simulink model "plotter_spring_damper"  (R2025a)
settings: Solver=VariableStepAuto  StartTime=0.0  StopTime=6  FixedStep=0.0001  MaxStep=1e-3  RelTol=1e-3
values from neighbouring files (symbols this model uses):
  alfa = cos(0.34906585)    [parameters.m]
  B_m = 0.000002    (= 2e-06)    [parameters.m]
  C = 3    [parameters.m]
  g = 9.8    [parameters.m]
  Gr = 1/30    (= 0.0333333333333)    [parameters.m]
  J_m = 0.000004    (= 4e-06)    [parameters.m]
  K = p_otimos(1)    [aproxima_segunda_ordem.m]    (also in motor_param.m = 23.26; parameters.m = 2040; valores_bruno.m = 23.26)
  K_t = 0.009    [parameters.m]
  L = 0.3    [cinematic_sim.m]    (also in parameters.m)
  L_a = 0.0023    [parameters.m]
  m = 0.1    [parameters.m]
  R = 0.017    [parameters.m]
  R_a = 2.182    [parameters.m]
libraries: slpidlib x2
settings Model: SimulationMode=accelerator  Creator=bruno  LastModifiedBy=bruno

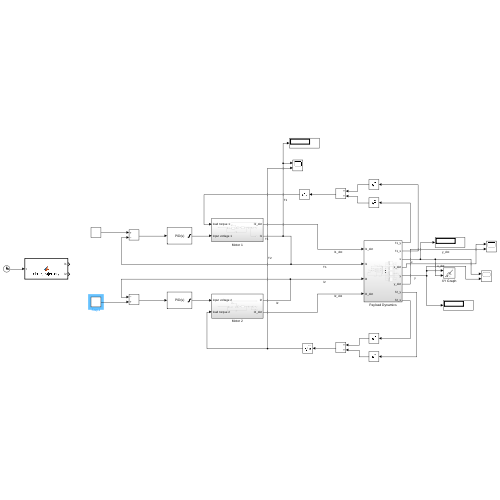
[thumbnail: Simulink's stored preview of the top-level diagram]
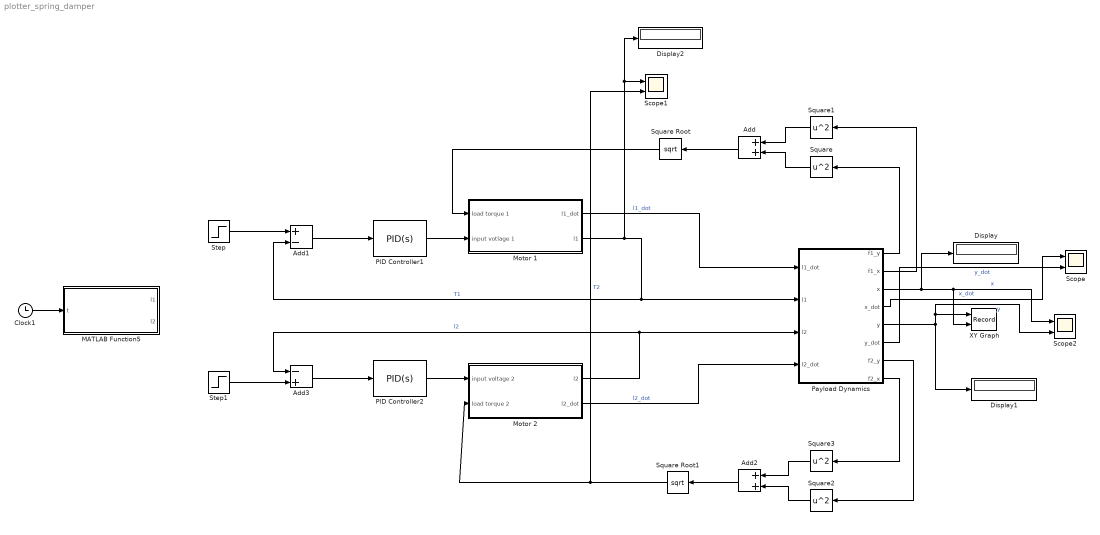
== system plotter_spring_damper ==
  Add : Sum
  Add1 : Sum  Inputs=+-
  Add2 : Sum
  Add3 : Sum  Inputs=-+
  Clock1 : Clock
      settings: Decimation=1000
  Display : Display
  Display1 : Display
  Display2 : Display
  MATLAB Function5 : MATLAB Function  TreatAsAtomicUnit=on
  Motor 1 : Subsystem
  Motor 2 : Subsystem
  PID Controller1 : slpidlib/PID Controller  Controller=PID  Form=Parallel  TimeDomain=Continuous-time  UseExternalTs=off  SampleTime=-1  IntegratorMethod=Forward Euler  FilterMethod=Forward Euler  ControllerParametersSource=internal  P=5109.01806071816  I=6474.67483762337  UseKiTs=off  D=175.0621895201  UseExternalDerivativeSource=off  N=17340.6505292231  UseFilter=on  TunerSelectOption=Transfer Function Based (PID Tuner App)  InitialConditionSource=internal  InitialConditionForIntegrator=0  InitialConditionForFilter=0  DifferentiatorICPrevScaledInput=0  ExternalReset=none  TrackingMode=off  Kt=1  LimitOutput=on  SatLimitsSource=internal  UpperSaturationLimit=12  LowerSaturationLimit=-12  LinearizeAsGain=on  AntiWindupMode=none  Kb=1  LimitIntegrator=off  UpperIntegratorSaturationLimit=inf  LowerIntegratorSaturationLimit=-inf  POutMin=[]  POutMax=[]  IOutMin=[]  IOutMax=[]  DOutMin=[]  DOutMax=[]  NOutMin=[]  NOutMax=[]  SumOutMin=[]  SumOutMax=[]  SaturationOutMin=[]  SaturationOutMax=[]  PParamMin=[]  PParamMax=[]  IParamMin=[]  IParamMax=[]  DParamMin=[]  DParamMax=[]  NParamMin=[]  NParamMax=[]  KbParamMin=[]  KbParamMax=[]  KtParamMin=[]  KtParamMax=[]  KbOutMin=[]  KbOutMax=[]  KtOutMin=[]  KtOutMax=[]  IntegratorOutMin=[]  IntegratorOutMax=[]  FilterOutMin=[]  FilterOutMax=[]  SumI1OutMin=[]  SumI1OutMax=[]  SumI2OutMin=[]  SumI2OutMax=[]  SumI3OutMin=[]  SumI3OutMax=[]  SumI4OutMin=[]  SumI4OutMax=[]  SumDOutMin=[]  SumDOutMax=[]  DifferentiatorOutMin=[]  DifferentiatorOutMax=[]  FilterDiffOutCoefMin=[]  FilterDiffOutCoefMax=[]  ReciprocalOutMin=[]  ReciprocalOutMax=[]  SumDenOutMin=[]  SumDenOutMax=[]  SumNumOutMin=[]  SumNumOutMax=[]  DivideOutMin=[]  DivideOutMax=[]  UdiffTsProdOutMin=[]  UdiffTsProdOutMax=[]  NTsProdOutMin=[]  NTsProdOutMax=[]  UintegralTsProdOutMin=[]  UintegralTsProdOutMax=[]  UngainTsProdOutMin=[]  UngainTsProdOutMax=[]  ClampingZeroOutDataTypeStr=Inherit: Inherit via back propagation  ClampingZeroOutMin=[]  ClampingZeroOutMax=[]  FilterDenConstantOutDataTypeStr=Inherit: Inherit via back propagation  FilterDenConstantOutMin=[]  FilterDenConstantOutMax=[]  PCopyOutDataTypeStr=Inherit: Inherit via back propagation  PCopyOutMin=[]  PCopyOutMax=[]  NCopyOutDataTypeStr=Inherit: Inherit via back propagation  NCopyOutMin=[]  NCopyOutMax=[]  IntegratorContinuousStateAttributes=''  IntegratorStateMustResolveToSignalObject=off  IntegratorRTWStateStorageClass=Auto  FilterContinuousStateAttributes=''  FilterStateMustResolveToSignalObject=off  FilterRTWStateStorageClass=Auto  ParallelPVariant=InternalParameters  IdealPVariant=Disabled  IVariant=InternalParameters  DVariant=InternalParameters  IntegratorVariant=Continuous  SatVariant=Enabled  AWVariant=Passthrough  PCopyVariant=Disabled  TRVariant=Disabled  FdbkBlocksVariant=Forward  IdealPFdbkVariant=Disabled  SatFdbkVariant=Disabled  DerivativeFilterVariant=ContFilter  NVariant=InternalParameters  NCopyVariant=Disabled  FilterICVariant=InternalICsFilter  IntegratorICVariant=InternalICs  ExternalResetVariant=Disabled  TRSumVariant=Passthrough  SumFdbkVariant=Disabled  SumVariant=Sum_PID  TsampFilterVariant=InternalTs  TsampNgainVariant=Passthrough  TsampIntegralVariant=Disabled_SignalSpec  ExternalSaturationOutDataTypeStr=Inherit: Same as second input  DerivativeSourceVariant=ErrorSignal  PreIntVariant=InternalPreInt
  PID Controller2 : slpidlib/PID Controller  Controller=PID  Form=Parallel  TimeDomain=Continuous-time  UseExternalTs=off  SampleTime=-1  IntegratorMethod=Forward Euler  FilterMethod=Forward Euler  ControllerParametersSource=internal  P=5109.01806071816  I=6474.67483762337  UseKiTs=off  D=175.0621895201  UseExternalDerivativeSource=off  N=17340.6505292231  UseFilter=on  TunerSelectOption=Transfer Function Based (PID Tuner App)  InitialConditionSource=internal  InitialConditionForIntegrator=0  InitialConditionForFilter=0  DifferentiatorICPrevScaledInput=0  ExternalReset=none  TrackingMode=off  Kt=1  LimitOutput=on  SatLimitsSource=internal  UpperSaturationLimit=12  LowerSaturationLimit=-12  LinearizeAsGain=on  AntiWindupMode=none  Kb=1  LimitIntegrator=off  UpperIntegratorSaturationLimit=inf  LowerIntegratorSaturationLimit=-inf  POutMin=[]  POutMax=[]  IOutMin=[]  IOutMax=[]  DOutMin=[]  DOutMax=[]  NOutMin=[]  NOutMax=[]  SumOutMin=[]  SumOutMax=[]  SaturationOutMin=[]  SaturationOutMax=[]  PParamMin=[]  PParamMax=[]  IParamMin=[]  IParamMax=[]  DParamMin=[]  DParamMax=[]  NParamMin=[]  NParamMax=[]  KbParamMin=[]  KbParamMax=[]  KtParamMin=[]  KtParamMax=[]  KbOutMin=[]  KbOutMax=[]  KtOutMin=[]  KtOutMax=[]  IntegratorOutMin=[]  IntegratorOutMax=[]  FilterOutMin=[]  FilterOutMax=[]  SumI1OutMin=[]  SumI1OutMax=[]  SumI2OutMin=[]  SumI2OutMax=[]  SumI3OutMin=[]  SumI3OutMax=[]  SumI4OutMin=[]  SumI4OutMax=[]  SumDOutMin=[]  SumDOutMax=[]  DifferentiatorOutMin=[]  DifferentiatorOutMax=[]  FilterDiffOutCoefMin=[]  FilterDiffOutCoefMax=[]  ReciprocalOutMin=[]  ReciprocalOutMax=[]  SumDenOutMin=[]  SumDenOutMax=[]  SumNumOutMin=[]  SumNumOutMax=[]  DivideOutMin=[]  DivideOutMax=[]  UdiffTsProdOutMin=[]  UdiffTsProdOutMax=[]  NTsProdOutMin=[]  NTsProdOutMax=[]  UintegralTsProdOutMin=[]  UintegralTsProdOutMax=[]  UngainTsProdOutMin=[]  UngainTsProdOutMax=[]  ClampingZeroOutDataTypeStr=Inherit: Inherit via back propagation  ClampingZeroOutMin=[]  ClampingZeroOutMax=[]  FilterDenConstantOutDataTypeStr=Inherit: Inherit via back propagation  FilterDenConstantOutMin=[]  FilterDenConstantOutMax=[]  PCopyOutDataTypeStr=Inherit: Inherit via back propagation  PCopyOutMin=[]  PCopyOutMax=[]  NCopyOutDataTypeStr=Inherit: Inherit via back propagation  NCopyOutMin=[]  NCopyOutMax=[]  IntegratorContinuousStateAttributes=''  IntegratorStateMustResolveToSignalObject=off  IntegratorRTWStateStorageClass=Auto  FilterContinuousStateAttributes=''  FilterStateMustResolveToSignalObject=off  FilterRTWStateStorageClass=Auto  ParallelPVariant=InternalParameters  IdealPVariant=Disabled  IVariant=InternalParameters  DVariant=InternalParameters  IntegratorVariant=Continuous  SatVariant=Enabled  AWVariant=Passthrough  PCopyVariant=Disabled  TRVariant=Disabled  FdbkBlocksVariant=Forward  IdealPFdbkVariant=Disabled  SatFdbkVariant=Disabled  DerivativeFilterVariant=ContFilter  NVariant=InternalParameters  NCopyVariant=Disabled  FilterICVariant=InternalICsFilter  IntegratorICVariant=InternalICs  ExternalResetVariant=Disabled  TRSumVariant=Passthrough  SumFdbkVariant=Disabled  SumVariant=Sum_PID  TsampFilterVariant=InternalTs  TsampNgainVariant=Passthrough  TsampIntegralVariant=Disabled_SignalSpec  ExternalSaturationOutDataTypeStr=Inherit: Same as second input  DerivativeSourceVariant=ErrorSignal  PreIntVariant=InternalPreInt
  Payload Dynamics : Subsystem
  Scope : Scope  NumInputPorts=2
      settings: ActiveDisplayYMinimum=-0.62327143885854985  ActiveDisplayYMaximum=0.35966972632216176
  Scope1 : Scope  NumInputPorts=2
      settings: ActiveDisplayYMinimum=-0.38341696076365567  ActiveDisplayYMaximum=3.450752646872902  DataLoggingVariableName=ScopeData2
  Scope2 : Scope  NumInputPorts=2
      settings: ActiveDisplayYMinimum=0.20131924623409117  ActiveDisplayYMaximum=0.42229314319938704  DataLoggingVariableName=ScopeData3
  Square{,1..3} (4 alike) : Math  Operator=square
  Square Root : Sqrt
  Square Root1 : Sqrt
  Step : Step  Time=0  After=0.43  SampleTime=0
  Step1 : Step  Time=0  After=0.36  SampleTime=0
  XY Graph : Record  NumPorts=2.0  FileSettingsInternal="{\"entries\":[{\"content\":{\"excelSettings\":{\"content\":{},\"type\":\"Streamout.ExcelSettings\"},\"parquetSettings\":{\"content\":{},\"type\":\"Streamout.ParquetSettings\"}},\"type\":\"Streamout.FileSettingStorage\",\"uuid\":\"\"}],\"packageUris\":[\"http:\\/\\/schema.mathworks.com\\/mf0\\/streamout_blocks\\/R2020a\"],\"version\":\"1.0\"}"  FrameSettings=[0, 0]  Layout=[1 1]  SignalsInternal="{\"entries\":[{\"content\":{\"signals\":[{\"content\":{\"blockPath\":[],\"dimensions\":[1],\"domain\":\"\",\"lineColor\":\"#a2142f\",\"plots\":[ 1 ],\"port\":1,\"signalID\":1,\"signalName\":\"y\"},\"type\":\"RecordBlkView.Signal\",\"uuid\":\"\"},{\"content\":{\"blockPath\":[],\"dimensions\":[1],\"domain\":\"\",\"lineColor\":\"#139fff\",\"plots\":[ 1 ],\"port\":2,\"signalID\":2,\"signalName\":\"x\"},\"type\":\"RecordBlkView.Signal\",\"uuid\":\"\"}]},\"type\":\"RecordBlkView.InputSignals\",\"uuid\":\"\"}],\"packageUris\":[\"http:\\/\\/schema.mathworks.com\\/mf0\\/streamout_blocks\\/R2020a\"],\"version\":\"1.0\"}"  VisualizationBindings="{\"xyplotplugin\":{\"info\":[{\"series\":[{\"bindingParametersList\":[{\"parameter\":\"X-Axis\",\"signalID\":1,\"signalName\":\"y\"},{\"parameter\":\"Y-Axis\",\"signalID\":2,\"signalName\":\"x\"}],\"seriesID\":0}],\"subplotID\":1}]}}"  CompatibilityTag=XY
  wires:
  Square1/1 -> Add/1
  Square/1 -> Add/2
  Add/1 -> Square Root/1
  Square2/1 -> Add2/2
  Add2/1 -> Square Root1/1
  Square3/1 -> Add2/1
  PID Controller2/1 -> Motor 2/1(input voltage 2)
  PID Controller1/1 -> Motor 1/2(input votlage 1)
  Payload Dynamics/8(f2_x) -> Square3/1
  Payload Dynamics/7(f2_y) -> Square2/1
  Add1/1 -> PID Controller1/1
  Add3/1 -> PID Controller2/1
  Payload Dynamics/2(f1_x) -> Square1/1
  Payload Dynamics/3(x) -> XY Graph/2, Scope2/1, Display/1  "x"
  Payload Dynamics/5(y) -> XY Graph/1, Scope2/2, Display1/1  "y"
  Payload Dynamics/1(f1_y) -> Square/1
  Motor 1/1(l1_dot) -> Payload Dynamics/1(l1_dot)  "l1_dot"
  Motor 1/2(l1) -> Display2/1, Scope1/1, Add1/2, Payload Dynamics/2(l1)  "T1"
  Motor 2/2(l2_dot) -> Payload Dynamics/4(l2_dot)  "l2_dot"
  Square Root/1 -> Motor 1/1(load torque 1)
  Square Root1/1 -> Scope1/2, Motor 2/2(load torque 2)  "T2"
  Motor 2/1(l2) -> Add3/1, Payload Dynamics/3(l2)  "l2"
  Clock1/1 -> MATLAB Function5/1(t)
  Payload Dynamics/4(x_dot) -> Scope/1  "x_dot"
  Payload Dynamics/6(y_dot) -> Scope/2  "y_dot"
  Step/1 -> Add1/1
  Step1/1 -> Add3/2

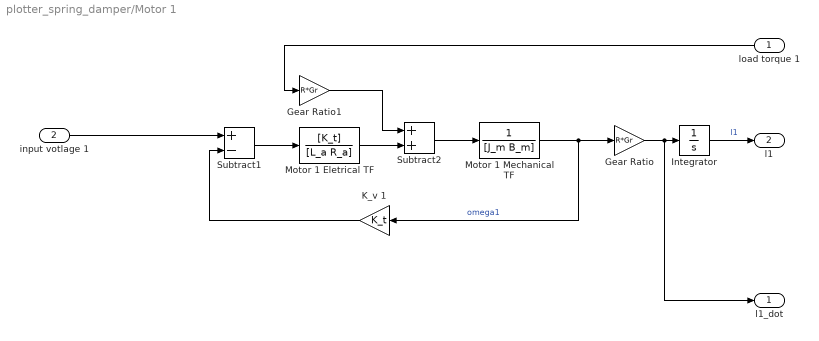
== system plotter_spring_damper/Motor 1 ==
  load torque 1 : Inport
  input votlage 1 : Inport  Port=2
  Gear Ratio : Gain  Gain=R*Gr
  Gear Ratio1 : Gain  Gain=R*Gr
  Integrator : Integrator  InitialCondition=0.461411
  K_v 1 : Gain  Gain=K_t
  Motor 1 Eletrical TF : TransferFcn  Numerator=[K_t]  Denominator=[L_a R_a]
  Motor 1 Mechanical TF : TransferFcn  Denominator=[J_m B_m]
  Subtract1 : Sum  Inputs=+-
  Subtract2 : Sum
  l1_dot : Outport
  l1 : Outport  Port=2
  wires:
  Motor 1 Eletrical TF/1 -> Subtract2/2
  load torque 1/1 -> Gear Ratio1/1
  K_v 1/1 -> Subtract1/2
  Gear Ratio1/1 -> Subtract2/1
  Subtract1/1 -> Motor 1 Eletrical TF/1
  Subtract2/1 -> Motor 1 Mechanical TF/1
  input votlage 1/1 -> Subtract1/1
  Motor 1 Mechanical TF/1 -> K_v 1/1, Gear Ratio/1  "omega1"
  Gear Ratio/1 -> l1_dot/1, Integrator/1
  Integrator/1 -> l1/1  "l1"

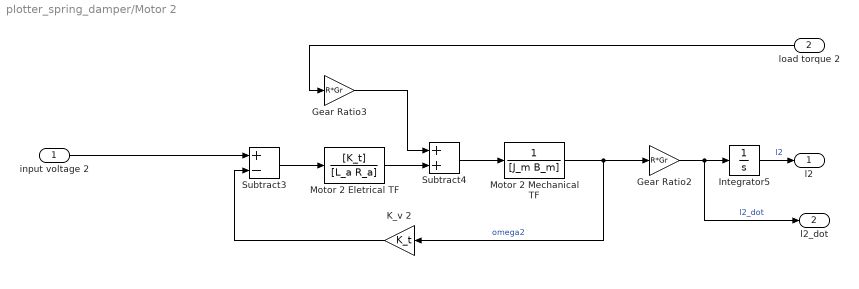
== system plotter_spring_damper/Motor 2 ==
  input voltage 2 : Inport
  load torque 2 : Inport  Port=2
  Gear Ratio2 : Gain  Gain=R*Gr
  Gear Ratio3 : Gain  Gain=R*Gr
  Integrator5 : Integrator  InitialCondition=0.406079
  K_v 2 : Gain  Gain=K_t
  Motor 2 Eletrical TF : TransferFcn  Numerator=[K_t]  Denominator=[L_a R_a]
  Motor 2 Mechanical TF : TransferFcn  Denominator=[J_m B_m]
  Subtract3 : Sum  Inputs=+-
  Subtract4 : Sum
  l2 : Outport
  l2_dot : Outport  Port=2
  wires:
  input voltage 2/1 -> Subtract3/1
  Motor 2 Eletrical TF/1 -> Subtract4/2
  Integrator5/1 -> l2/1  "l2"
  Subtract3/1 -> Motor 2 Eletrical TF/1
  Gear Ratio3/1 -> Subtract4/1
  Subtract4/1 -> Motor 2 Mechanical TF/1
  load torque 2/1 -> Gear Ratio3/1
  K_v 2/1 -> Subtract3/2
  Gear Ratio2/1 -> l2_dot/1, Integrator5/1  "l2_dot"
  Motor 2 Mechanical TF/1 -> Gear Ratio2/1, K_v 2/1  "omega2"

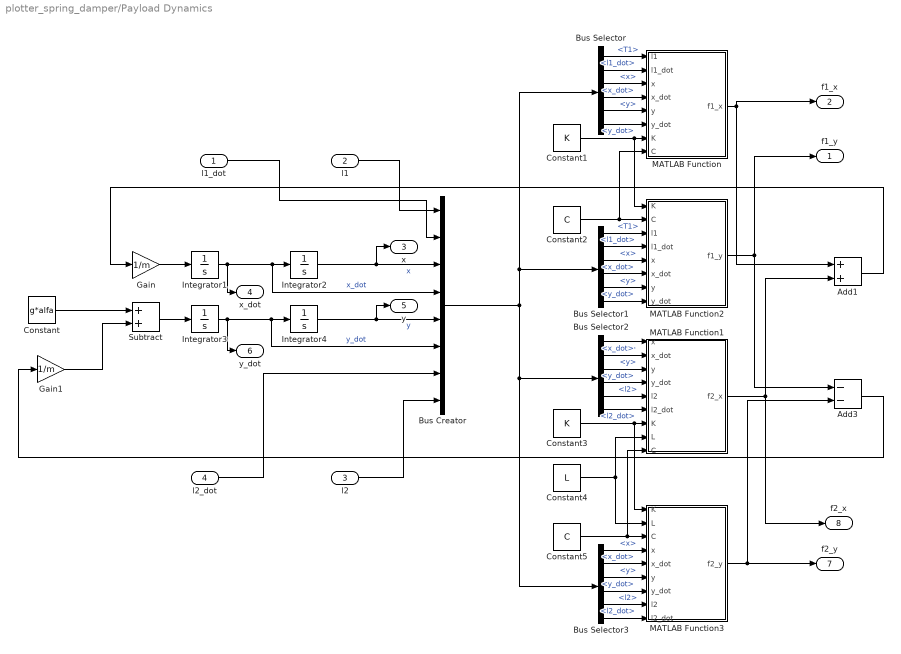
== system plotter_spring_damper/Payload Dynamics ==
  l1_dot : Inport
  l1 : Inport  Port=2
  l2 : Inport  Port=3
  l2_dot : Inport  Port=4
  Add1 : Sum
  Add3 : Sum  Inputs=--
  Bus Creator : BusCreator  Inputs=8
  Bus Selector : BusSelector  OutputSignals=T1,l1_dot,x,x_dot,y,y_dot
  Bus Selector1 : BusSelector  OutputSignals=T1,l1_dot,x,x_dot,y,y_dot
  Bus Selector2 : BusSelector  OutputSignals=x,x_dot,y,y_dot,l2,l2_dot
  Bus Selector3 : BusSelector  OutputSignals=x,x_dot,y,y_dot,l2,l2_dot
  Constant : Constant  Value=g*alfa
  Constant1 : Constant  Value=K
  Constant2 : Constant  Value=C
  Constant3 : Constant  Value=K
  Constant4 : Constant  Value=L
  Constant5 : Constant  Value=C
  Gain : Gain  Gain=1/m
  Gain1 : Gain  Gain=1/m
  Integrator1 : Integrator
  Integrator2 : Integrator  InitialCondition=0.23
  Integrator3 : Integrator
  Integrator4 : Integrator  InitialCondition=0.4
  MATLAB Function : MATLAB Function  TreatAsAtomicUnit=on
  MATLAB Function1 : MATLAB Function  TreatAsAtomicUnit=on
  MATLAB Function2 : MATLAB Function  TreatAsAtomicUnit=on
  MATLAB Function3 : MATLAB Function  TreatAsAtomicUnit=on
  Subtract : Sum
  f1_y : Outport
  f1_x : Outport  Port=2
  x : Outport  Port=3
  x_dot : Outport  Port=4
  y : Outport  Port=5
  y_dot : Outport  Port=6
  f2_y : Outport  Port=7
  f2_x : Outport  Port=8
  wires:
  Bus Selector1/2 -> MATLAB Function2/4(l1_dot)  "<l1_dot>"
  Bus Selector1/1 -> MATLAB Function2/3(l1)  "<T1>"
  Add3/1 -> Gain1/1
  Bus Selector1/6 -> MATLAB Function2/8(y_dot)  "<y_dot>"
  Constant3/1 -> MATLAB Function3/1(K), MATLAB Function1/7(K)
  Bus Selector1/4 -> MATLAB Function2/6(x_dot)  "<x_dot>"
  Bus Selector/4 -> MATLAB Function/4(x_dot)  "<x_dot>"
  Bus Selector/2 -> MATLAB Function/2(l1_dot)  "<l1_dot>"
  Bus Selector/1 -> MATLAB Function/1(l1)  "<T1>"
  Bus Selector/6 -> MATLAB Function/6(y_dot)  "<y_dot>"
  Bus Selector/3 -> MATLAB Function/3(x)  "<x>"
  Bus Selector/5 -> MATLAB Function/5(y)  "<y>"
  Integrator1/1 -> Bus Creator/4, Integrator2/1, x_dot/1  "x_dot"
  Constant/1 -> Subtract/1
  Bus Selector2/5 -> MATLAB Function1/5(l2)  "<l2>"
  Constant5/1 -> MATLAB Function3/3(C), MATLAB Function1/9(C)
  Integrator3/1 -> y_dot/1, Bus Creator/6, Integrator4/1  "y_dot"
  Bus Selector3/1 -> MATLAB Function3/4(x)  "<x>"
  Bus Selector3/3 -> MATLAB Function3/6(y)  "<y>"
  Constant4/1 -> MATLAB Function1/8(L), MATLAB Function3/2(L)
  Add1/1 -> Gain/1
  l1_dot/1 -> Bus Creator/2
  MATLAB Function/1(f1_x) -> Add1/1, f1_x/1
  l2_dot/1 -> Bus Creator/7
  l2/1 -> Bus Creator/8
  Bus Selector2/3 -> MATLAB Function1/3(y)  "<y>"
  Constant1/1 -> MATLAB Function2/1(K), MATLAB Function/7(K)
  l1/1 -> Bus Creator/1
  MATLAB Function3/1(f2_y) -> Add3/2, f2_y/1
  Gain/1 -> Integrator1/1
  Bus Selector2/1 -> MATLAB Function1/1(x)  "<x>"
  MATLAB Function1/1(f2_x) -> f2_x/1, Add1/2
  Bus Selector2/2 -> MATLAB Function1/2(x_dot)  "<x_dot>"
  Bus Selector3/6 -> MATLAB Function3/9(l2_dot)  "<l2_dot>"
  Integrator4/1 -> y/1, Bus Creator/5  "y"
  Bus Selector2/4 -> MATLAB Function1/4(y_dot)  "<y_dot>"
  Integrator2/1 -> x/1, Bus Creator/3  "x"
  Bus Creator/1 -> Bus Selector3/1, Bus Selector2/1, Bus Selector1/1, Bus Selector/1
  Bus Selector3/5 -> MATLAB Function3/8(l2)  "<l2>"
  MATLAB Function2/1(f1_y) -> f1_y/1, Add3/1
  Bus Selector3/4 -> MATLAB Function3/7(y_dot)  "<y_dot>"
  Bus Selector3/2 -> MATLAB Function3/5(x_dot)  "<x_dot>"
  Constant2/1 -> MATLAB Function2/2(C), MATLAB Function/8(C)
  Subtract/1 -> Integrator3/1
  Bus Selector1/3 -> MATLAB Function2/5(x)  "<x>"
  Bus Selector1/5 -> MATLAB Function2/7(y)  "<y>"
  Gain1/1 -> Subtract/2
  Bus Selector2/6 -> MATLAB Function1/6(l2_dot)  "<l2_dot>"

== matlab function plotter_spring_damper/Payload Dynamics/MATLAB Function1 ==
  data: x input; x_dot input; f2_x output; y input; y_dot input; l2 input; l2_dot input; K input; L input; C input
function f2_x = F2_x(x,x_dot,y,y_dot,l2,l2_dot,K,L,C)
    distance2 = sqrt((L-x)^2 + y^2);
    if distance2 > l2 
        f2_x = (K*(distance2 -l2) + C*((x*x_dot -L*x_dot + y*y_dot)/distance2 - l2_dot))*(L-x)/distance2;
    else
        f2_x = 0;
    end
end

== matlab function plotter_spring_damper/Payload Dynamics/MATLAB Function ==
  data: l1 input; l1_dot input; x input; x_dot input; f1_x output; y input; y_dot input; K input; C input
function f1_x = F1_x(l1,l1_dot,x,x_dot,y,y_dot,K,C)
    distance1 = sqrt(x^2+y^2);
    if distance1 > l1
        f1_x = (K*(-distance1 + l1) + C*(-(x*x_dot + y*y_dot)/distance1 + l1_dot))*x/distance1;
    else
        f1_x = 0;
    end
end

== matlab function plotter_spring_damper/Payload Dynamics/MATLAB Function2 ==
  data: K input; C input; l1 input; l1_dot input; x input; x_dot input; f1_y output; y input; y_dot input
function f1_y = F1_y(K,C,l1,l1_dot,x,x_dot,y,y_dot)
    distance1 = sqrt(x^2+y^2);
    if distance1 > l1 
        f1_y = (K*(distance1 - l1) +  C*((x*x_dot + y*y_dot)/distance1 - l1_dot))*abs(y)/distance1;
    else
        f1_y = 0;
    end
end

== matlab function plotter_spring_damper/Payload Dynamics/MATLAB Function3 ==
  data: K input; L input; C input; x input; x_dot input; y input; y_dot input; l2 input; f2_y output; l2_dot input
function f2_y = F2_y(K,L,C,x,x_dot,y,y_dot,l2,l2_dot)
    distance2 = sqrt((L-x)^2 + y^2);
    if distance2 > l2 
        f2_y = (K*(distance2 -l2) + C*((x*x_dot -L*x_dot + y*y_dot)/distance2 - l2_dot))*abs(y)/distance2;
    else
        f2_y = 0;
    end
end

== matlab function plotter_spring_damper/MATLAB Function5 ==
  data: l1 output; l2 output; t input
function [l1, l2] = circle_trajectory(t)
% Generate (x, y) circular trajectory given time t

% Parameters
T = 6;           % Period (seconds)
r = 0.08;        % Radius (meters)
x0 = 0.15;       % Center x (meters)
y0 = 0.4;        % Center y (meters)
L = 0.3;

% Equations
angle = 2 * pi * t / T;
x = r * cos(angle) + x0;
y = r * sin(angle) + y0;
l1 = sqrt(x^2 + y^2);
l2 = sqrt((L - x)^2 + y^2);
